simulink model "CToSimulink_V1"  (R2021a)
settings: Solver=FixedStepAuto  StartTime=0.0  StopTime=inf  RelTol=1e-3
libraries: vexcommonlib x4, vexarmcortexlib x4
settings Model: ExtModeTrigDuration=25  Creator=Mihai Nicoara  LastModifiedBy=Mihai Nicoara
settings OptimizationCC: EnhancedBackFolding=on  PassReuseOutputArgsAs=Individual arguments  ZeroExternalMemoryAtStartup=off  ZeroInternalMemoryAtStartup=off  MaxStackSize=64  OptimizeBlockOrder=speed  DifferentSizesBufferReuse=on  OptimizationCustomize=off  EfficientTunableParamExpr=on
settings DebuggingCC: ParameterTunabilityLossMsg=error
settings HardwareCC: ProdBitPerPointer=32  ProdBitPerSizeT=32  ProdBitPerPtrDiffT=32  ProdLargestAtomicInteger=Long  ProdLargestAtomicFloat=Double  ProdWordSize=32  ProdHWDeviceType=ARM Compatible->ARM Cortex
settings SFSimCC: MATLABDynamicMemAlloc=off  SimTargetLang=C++
settings RTWCC: SystemTargetFile=ert.tlc  HardwareBoard=ARM Cortex-based VEX Microcontroller  TLCOptions="-aInlineSetEventsForThisBaseRateFcn=TLC_FALSE -aSuppressMultiTaskScheduler=TLC_FALSE  -aRateBasedStepFcn=0"  TemplateMakefile=ert_default_tmf  Toolchain=GNU Tools for VEX ARM Cortex
settings CodeAppCC: ForceParamTrailComments=on  IgnoreCustomStorageClasses=off  OperatorAnnotations=on  SimulinkDataObjDesc=on  SFDataObjDesc=on  InsertBlockDesc=on
settings ERTTargetCC: ExtModeTransport=1  ExtModeMexFile=ext_serial_win32_comm

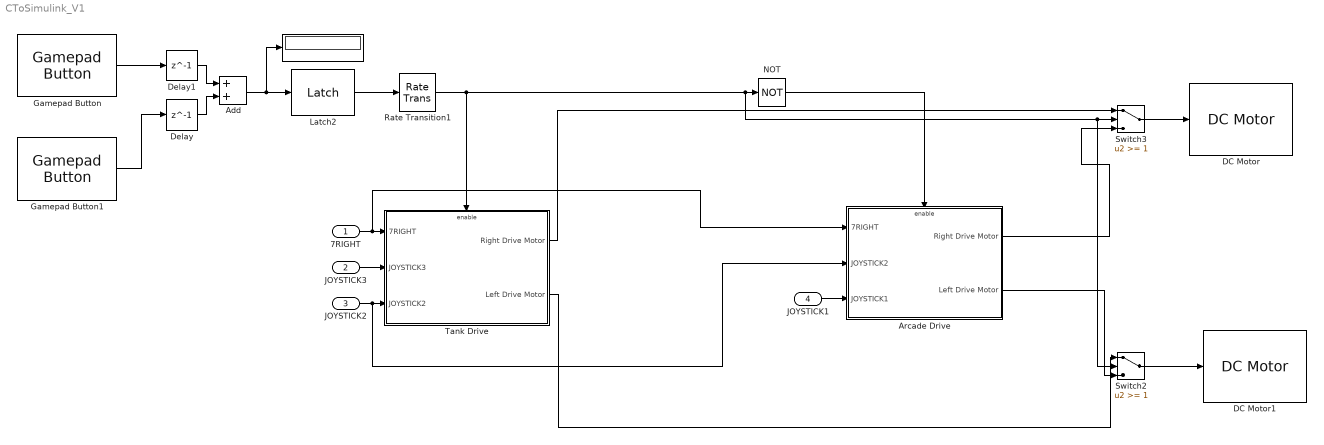
== system CToSimulink_V1 ==
  7RIGHT : Inport
  JOYSTICK3 : Inport  Port=2
  JOYSTICK2 : Inport  Port=3
  JOYSTICK1 : Inport  Port=4
  " " : Display
  Add : Sum
  "Arcade Drive " : Subsystem  TreatAsAtomicUnit=on
  DC Motor : vexarmcortexlib/Actuators/DC Motor  motor=2  scaleFactor=1/13.5  SimulationOut=off
      settings: SourceProductBaseCode=EC_VEX_MICRO
  DC Motor1 : vexarmcortexlib/Actuators/DC Motor  motor=9  scaleFactor=1/13.5  SimulationOut=off
      settings: SourceProductBaseCode=EC_VEX_MICRO
  Delay : Delay  DelayLength=1  InitialCondition=0  SampleTime=0.5
  Delay1 : Delay  DelayLength=1  InitialCondition=0  SampleTime=0.5
  Gamepad Button : vexarmcortexlib/Gamepad/Gamepad Button  joystick=1  chan=7  button56=Up  button78=Down  SimulationIn=off  SampleTime=0.02
      settings: SourceProductBaseCode=EC_VEX_MICRO
  Gamepad Button1 : vexarmcortexlib/Gamepad/Gamepad Button  joystick=1  chan=8  button56=Up  button78=Down  SimulationIn=off  SampleTime=0.02
      settings: SourceProductBaseCode=EC_VEX_MICRO
  Latch2 : vexcommonlib/Latch  output0=off  BlockPlatform=vexarmcortex
      settings: SourceProductBaseCode=EC_VEX_MICRO,VEXV5
  NOT : Logic  Operator=NOT  IconShape=distinctive  AllPortsSameDT=off  OutDataTypeStr=boolean
  Rate Transition1 : RateTransition  OutPortSampleTime=0.002
  Switch2 : Switch  Threshold=1
  Switch3 : Switch  Threshold=1
  "Tank Drive " : Subsystem  TreatAsAtomicUnit=on
  wires:
  "Tank Drive "/1(Right Drive Motor) -> Switch3/1
  JOYSTICK1/1 -> "Arcade Drive "/3(JOYSTICK1)
  Latch2/1 -> Rate Transition1/1
  "Tank Drive "/2(Left Drive Motor) -> Switch2/1
  "Arcade Drive "/1(Right Drive Motor) -> Switch3/3
  Add/1 -> " "/1, Latch2/1
  NOT/1 -> "Arcade Drive "/Enable
  7RIGHT/1 -> "Tank Drive "/1(7RIGHT), "Arcade Drive "/1(7RIGHT)
  JOYSTICK2/1 -> "Tank Drive "/3(JOYSTICK2), "Arcade Drive "/2(JOYSTICK2)
  "Arcade Drive "/2(Left Drive Motor) -> Switch2/3
  Delay1/1 -> Add/1
  Rate Transition1/1 -> NOT/1, Switch2/2, Switch3/2, "Tank Drive "/Enable
  Delay/1 -> Add/2
  JOYSTICK3/1 -> "Tank Drive "/2(JOYSTICK3)
  Switch3/1 -> DC Motor/1
  Switch2/1 -> DC Motor1/1
  Gamepad Button1/1 -> Delay/1
  Gamepad Button/1 -> Delay1/1

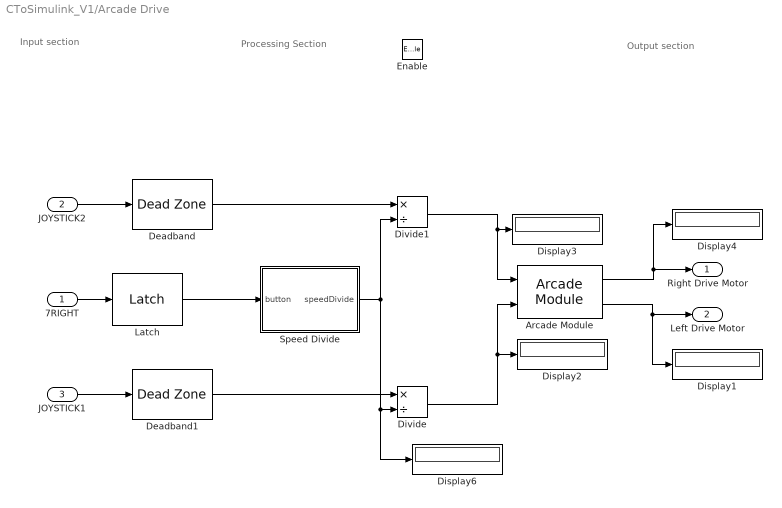
== system CToSimulink_V1/Arcade Drive  ==
  note: Output section
  note: Processing Section
  note: Input section
  7RIGHT : Inport
  JOYSTICK2 : Inport  Port=2
  JOYSTICK1 : Inport  Port=3
  Enable : EnablePort
  Arcade Module : vexcommonlib/Arcade Module  BlockPlatform=vexarmcortex
      settings: SourceProductBaseCode=EC_VEX_MICRO,VEXV5
  Deadband : DeadZone  LowerValue=-9  UpperValue=9  SaturateOnIntegerOverflow=on
  Deadband1 : DeadZone  LowerValue=-9  UpperValue=9  SaturateOnIntegerOverflow=on
  Display{1..4,6} (5 alike) : Display
  Divide : Product  Inputs=*/
  Divide1 : Product  Inputs=*/
  Latch : vexcommonlib/Latch  output0=off  BlockPlatform=vexarmcortex
      settings: SourceProductBaseCode=EC_VEX_MICRO,VEXV5
  Speed Divide : Stateflow chart  TreatAsAtomicUnit=on
  Right Drive Motor : Outport
  Left Drive Motor : Outport  Port=2
  wires:
  7RIGHT/1 -> Latch/1
  Speed Divide/1(speedDivide) -> Display6/1, Divide/2, Divide1/2
  Divide/1 -> Arcade Module/2, Display2/1
  Divide1/1 -> Arcade Module/1, Display3/1
  Arcade Module/1 -> Display4/1, Right Drive Motor/1
  Arcade Module/2 -> Display1/1, Left Drive Motor/1
  Latch/1 -> Speed Divide/1(button)
  JOYSTICK2/1 -> Deadband/1
  JOYSTICK1/1 -> Deadband1/1
  Deadband/1 -> Divide1/1
  Deadband1/1 -> Divide/1

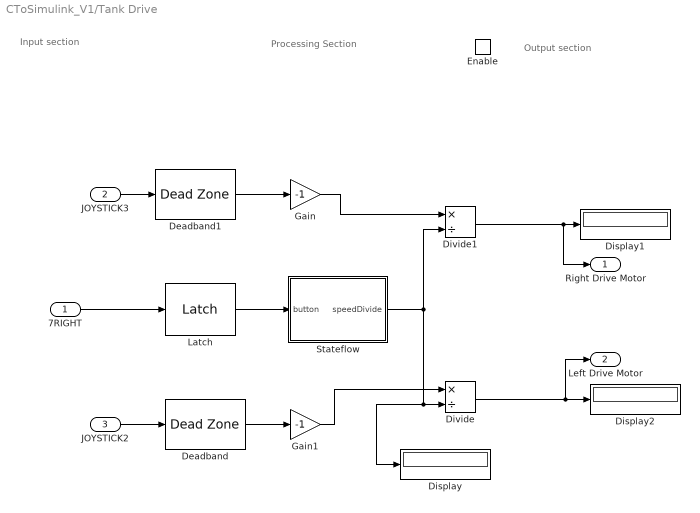
== system CToSimulink_V1/Tank Drive  ==
  note: Output section
  note: Processing Section
  note: Input section
  7RIGHT : Inport
  JOYSTICK3 : Inport  Port=2
  JOYSTICK2 : Inport  Port=3
  Enable : EnablePort
  Deadband : DeadZone  LowerValue=-9  UpperValue=9  SaturateOnIntegerOverflow=on
  Deadband1 : DeadZone  LowerValue=-9  UpperValue=9  SaturateOnIntegerOverflow=on
  Display : Display
  Display1 : Display
  Display2 : Display
  Divide : Product  Inputs=*/
  Divide1 : Product  Inputs=*/
  Gain : Gain  Gain=-1
  Gain1 : Gain  Gain=-1
  Latch : vexcommonlib/Latch  output0=off  BlockPlatform=vexarmcortex
      settings: SourceProductBaseCode=EC_VEX_MICRO,VEXV5
  Stateflow : Stateflow chart  TreatAsAtomicUnit=on
  Right Drive Motor : Outport
  Left Drive Motor : Outport  Port=2
  wires:
  7RIGHT/1 -> Latch/1
  Latch/1 -> Stateflow/1(button)
  Stateflow/1(speedDivide) -> Divide1/2, Display/1, Divide/2
  JOYSTICK3/1 -> Deadband1/1
  Divide1/1 -> Display1/1, Right Drive Motor/1
  Divide/1 -> Display2/1, Left Drive Motor/1
  JOYSTICK2/1 -> Deadband/1
  Gain/1 -> Divide1/1
  Gain1/1 -> Divide/1
  Deadband1/1 -> Gain/1
  Deadband/1 -> Gain1/1

== stateflow chart CToSimulink_V1/Arcade Drive /Speed Divide ==
  state Full_Speed
    entry:
    speedDivide = 1
  state Slow_Speed
    entry:
    speedDivide = 2
  (default) -> Full_Speed
  Full_Speed -> Slow_Speed : [button == 1]
  Slow_Speed -> Full_Speed : [button == 0]
  data: speedDivide output; button input

== stateflow chart CToSimulink_V1/Tank Drive /Stateflow ==
  state Full_Speed
    entry:
    speedDivide = 1
  state Slow_Speed
    entry:
    speedDivide = 2
  (default) -> Full_Speed
  Full_Speed -> Slow_Speed : [button]
  Slow_Speed -> Full_Speed : [button == 0]
  data: speedDivide output; button input
